simulink model "ZV_synthesis"  (R2018b)
settings: Solver=VariableStepAuto  StartTime=0.0  StopTime=0.05  MaxStep=1e-6  RelTol=1e-8
settings Model: Creator=secklesa  LastModifiedBy=secklesa

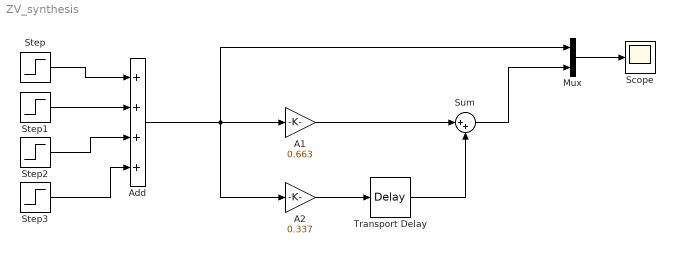
== system ZV_synthesis ==
  A1 : Gain  Gain=0.663
  A2 : Gain  Gain=0.337
  Add : Sum  Inputs=++++
  Mux : Mux  Inputs=2
  Scope : Scope
  Step : Step  Time=5E-3  SampleTime=0
  Step1 : Step  Time=15E-3  SampleTime=0
  Step2 : Step  Time=25E-3  After=-1  SampleTime=0
  Step3 : Step  Time=35E-3  After=-1  SampleTime=0
  Sum : Sum  Inputs=|++
  Transport Delay : TransportDelay  DelayTime=0.001
  wires:
  Step2/1 -> Add/3
  Step1/1 -> Add/2
  Step3/1 -> Add/4
  Step/1 -> Add/1
  Add/1 -> Mux/1, A2/1, A1/1
  Mux/1 -> Scope/1
  A1/1 -> Sum/1
  Sum/1 -> Mux/2
  A2/1 -> Transport Delay/1
  Transport Delay/1 -> Sum/2
